simulink model "allocation_test"  (R2022b)
settings: Solver=VariableStepAuto  StartTime=0.0  StopTime=10.0  RelTol=1e-3
libraries: MarineRoboticsLib x1
settings Model: Creator=dnad  LastModifiedBy=dnad

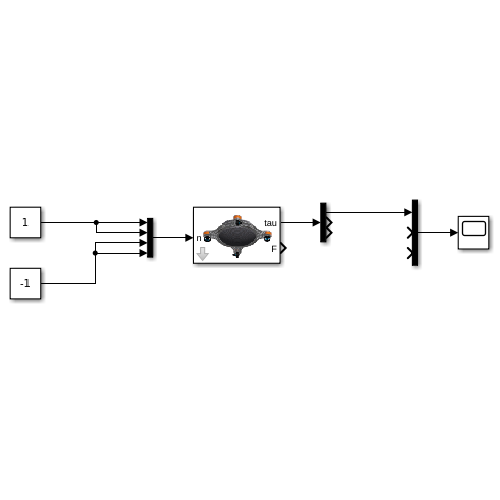
[thumbnail: Simulink's stored preview of the top-level diagram]
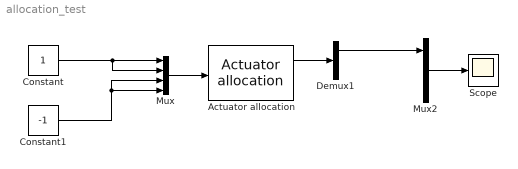
== system allocation_test ==
  Actuator allocation : MarineRoboticsLib/Actuator allocation  Tm=0  B="[0.25, 0.25, -0.25, -0.25; -0.25,  0.25, -0.25,  0.25; -0.25, 0.25, 0.25, -0.25]"  Keff=[1,1,1,1]
  Constant : Constant
  Constant1 : Constant  Value=-1
  Demux1 : Demux  Outputs=3
  Mux : Mux
  Mux2 : Mux  Inputs=3
  Scope : Scope
  wires:
  Mux/1 -> Actuator allocation/1
  Mux2/1 -> Scope/1
  Demux1/1 -> Mux2/1
  Constant/1 -> Mux/2, Mux/1
  Constant1/1 -> Mux/4, Mux/3
  Actuator allocation/1 -> Demux1/1
